simulink model "Assignment_II_simulink"  (R2024b)
settings: Solver=FixedStepAuto  StartTime=0.0  StopTime=inf  FixedStep=1/f_cmd  RelTol=1e-3
values from neighbouring files (symbols this model uses):
  ang_max = 0.05    [Assignment_II.m]
  dist_max = 0.01    [Assignment_II.m]
  k_v = 3    [Assignment_II.m]
  k_w_direction = 3    [Assignment_II.m]
  k_w_heading = 1    [Assignment_II.m]
  turtlebot3 = [ ... (first row only)    [Assignment_II.m]
  v_max = 0.2    [Assignment_II.m]
  yaw_rate_max = 0.4    [Assignment_II.m]
undefined symbols (not defined in the file or in its folder): Angular, Linear
libraries: robotlib x3, simulink x2
settings Model: PacingRate=20  Creator=vigno  LastModifiedBy=vigno
settings OptimizationCC: EnhancedBackFolding=on  PassReuseOutputArgsAs=Individual arguments  ZeroExternalMemoryAtStartup=off  ZeroInternalMemoryAtStartup=off  MaxStackSize=64  OptimizeBlockOrder=speed  DifferentSizesBufferReuse=on  OptimizationCustomize=off  EfficientTunableParamExpr=on
settings DebuggingCC: ParameterTunabilityLossMsg=error
settings HardwareCC: ProdBitPerPointer=32  ProdBitPerSizeT=32  ProdBitPerPtrDiffT=32  ProdLargestAtomicFloat=None  ProdIntDivRoundTo=Undefined  ProdEndianess=Unspecified  ProdWordSize=32  ProdHWDeviceType=Generic->Unspecified (assume 32-bit Generic)
settings ModelReferenceCC: EnableRefExpFcnMdlSchedulingChecks=on
settings SFSimCC: MATLABDynamicMemAlloc=off
settings RTWCC: Description=Embedded Coder  SystemTargetFile=ert.tlc  HardwareBoard=Robot Operating System (ROS)  TLCOptions="-aInlineSetEventsForThisBaseRateFcn=TLC_FALSE -aSuppressMultiTaskScheduler=TLC_FALSE  -aRateBasedStepFcn=0"  TemplateMakefile=ert_default_tmf  Toolchain=Catkin  TargetLang=C++  GPUComputeCapability=3.5
settings CodeAppCC: ForceParamTrailComments=on  IgnoreCustomStorageClasses=off  OperatorAnnotations=on  SimulinkDataObjDesc=on  SFDataObjDesc=on  InsertBlockDesc=on
settings ERTTargetCC: InlinedParameterPlacement=Hierarchical  DynamicArrayContainerType=coder::array

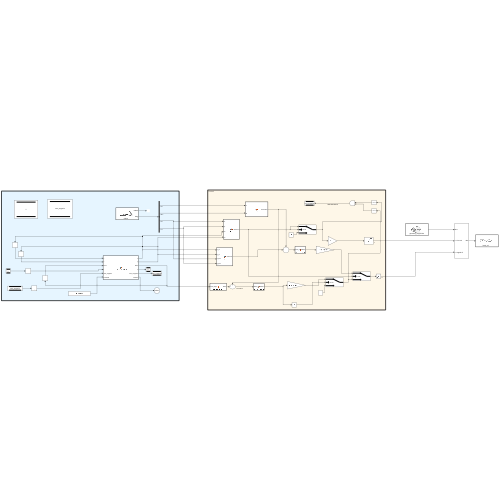
[thumbnail: Simulink's stored preview of the top-level diagram]
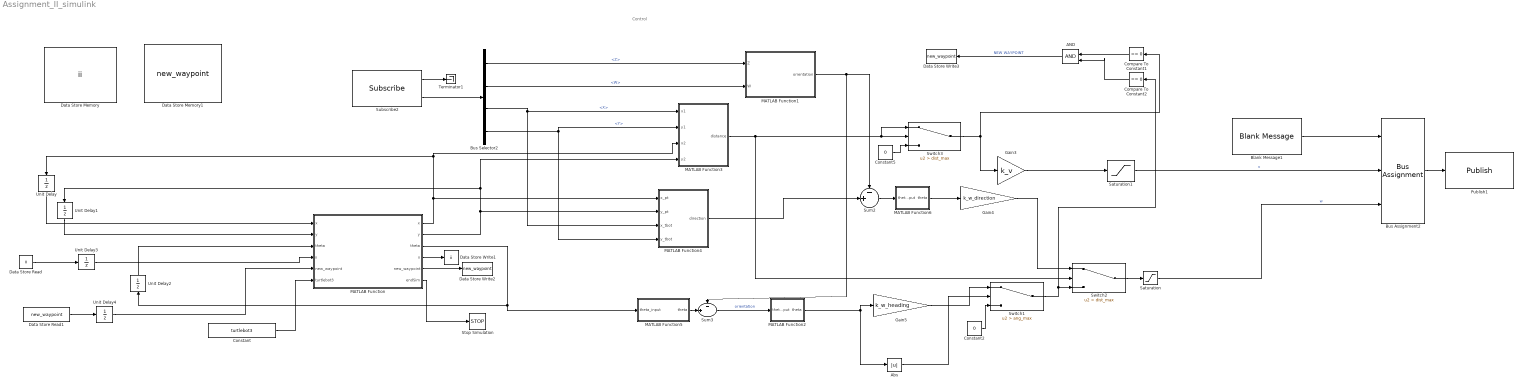
== system Assignment_II_simulink ==
  note: Control
  AND : Logic  IconShape=distinctive  AllPortsSameDT=off  OutDataTypeStr=boolean
  Abs : Abs  SaturateOnIntegerOverflow=off
  Blank Message1 : robotlib/Blank Message  messageClass=Message  entityType=geometry_msgs/Twist  messageType=geometry_msgs/Twist  SampleTime=-1  legacyBusStruct=off
  Bus Assignment2 : BusAssignment  AssignedSignals=Linear.X,Angular.Z
  Bus Selector2 : BusSelector  OutputSignals=Pose.Pose.Orientation.Z,Pose.Pose.Orientation.W,Pose.Pose.Position.X,Pose.Pose.Position.Y
  Compare To Constant1 : simulink/Logic and Bit Operations/Compare To Constant  relop===  const=0  OutDataTypeStr=boolean
  Compare To Constant2 : simulink/Logic and Bit Operations/Compare To Constant  relop===  const=0  OutDataTypeStr=boolean
  Constant : Constant  Value=turtlebot3
  Constant2 : Constant  Value=0
  Constant5 : Constant  Value=0
  Data Store Memory : DataStoreMemory  DataStoreName=ii  WriteAfterWriteMsg=warning  ShowAdditionalParam=off  OutDataTypeStr=double
  Data Store Memory1 : DataStoreMemory  DataStoreName=new_waypoint  WriteAfterWriteMsg=warning  ShowAdditionalParam=off
  Data Store Read : DataStoreRead  DataStoreName=ii  IndexOptions=Index vector (dialog)  Indices=1  OutputSizes=1
  Data Store Read1 : DataStoreRead  DataStoreName=new_waypoint  IndexOptions=Index vector (dialog)  Indices=1  OutputSizes=1
  Data Store Write1 : DataStoreWrite  DataStoreName=ii  IndexOptions=Index vector (dialog)  Indices=1  OutputSizes=1
  Data Store Write2 : DataStoreWrite  DataStoreName=new_waypoint  IndexOptions=Index vector (dialog)  Indices=1  OutputSizes=1
  Data Store Write3 : DataStoreWrite  DataStoreName=new_waypoint  IndexOptions=Index vector (dialog)  Indices=1  OutputSizes=1
  Gain3 : Gain  Gain=k_v
  Gain4 : Gain  Gain=k_w_direction
  Gain5 : Gain  Gain=k_w_heading
  MATLAB Function : MATLAB Function  TreatAsAtomicUnit=on
  MATLAB Function1 : MATLAB Function  TreatAsAtomicUnit=on
  MATLAB Function2 : MATLAB Function  TreatAsAtomicUnit=on
  MATLAB Function3 : MATLAB Function  TreatAsAtomicUnit=on
  MATLAB Function4 : MATLAB Function  TreatAsAtomicUnit=on
  MATLAB Function5 : MATLAB Function  TreatAsAtomicUnit=on
  MATLAB Function6 : MATLAB Function  TreatAsAtomicUnit=on
  Publish1 : robotlib/Publish  topicSource=Select from ROS network  topic=/cmd_vel  messageType=geometry_msgs/Twist  legacyBusStruct=off  messageQueueLength=1
  Saturation : Saturate  UpperLimit=yaw_rate_max  LowerLimit=- yaw_rate_max
  Saturation1 : Saturate  UpperLimit=v_max  LowerLimit=- v_max
  Stop Simulation : Stop
  Subscribe2 : robotlib/Subscribe  topicSource=Select from ROS network  topic=/odom  messageType=nav_msgs/Odometry  SampleTime=-1  legacyBusStruct=off  messageQueueLength=1
  Sum2 : Sum  Inputs=-+|
  Sum3 : Sum  Inputs=-+|
  Switch1 : Switch  Criteria=u2 > Threshold  Threshold=ang_max  SaturateOnIntegerOverflow=off  InputSameDT=off
  Switch2 : Switch  Criteria=u2 > Threshold  Threshold=dist_max  SaturateOnIntegerOverflow=off  InputSameDT=off
  Switch3 : Switch  Criteria=u2 > Threshold  Threshold=dist_max  SaturateOnIntegerOverflow=off  InputSameDT=off
  Terminator1 : Terminator
  Unit Delay{,1..4} (5 alike) : UnitDelay  SampleTime=-1  HasFrameUpgradeWarning=on
  wires:
  Subscribe2/2 -> Bus Selector2/1
  Blank Message1/1 -> Bus Assignment2/1
  Switch3/1 -> Compare To Constant1/1, Gain3/1
  Bus Selector2/2 -> MATLAB Function1/2(W)  "<W>"
  Gain3/1 -> Saturation1/1
  Bus Assignment2/1 -> Publish1/1
  Subscribe2/1 -> Terminator1/1
  Gain4/1 -> Switch2/1
  MATLAB Function4/1(direction) -> Sum2/2
  MATLAB Function3/1(distance) -> Switch3/1, Switch3/2, Switch2/2
  Constant5/1 -> Switch3/3
  Sum3/1 -> MATLAB Function2/1(theta_input)  "orientation"
  MATLAB Function1/1(orientation) -> Sum2/1, Sum3/1
  Bus Selector2/4 -> MATLAB Function3/2(y1), MATLAB Function4/4(y_tbot)  "<Y>"
  Bus Selector2/1 -> MATLAB Function1/1(Z)  "<Z>"
  Sum2/1 -> MATLAB Function6/1(theta_input)
  Bus Selector2/3 -> MATLAB Function4/3(x_tbot), MATLAB Function3/1(x1)  "<X>"
  AND/1 -> Data Store Write3/1  "NEW WAYPOINT"
  Data Store Read/1 -> Unit Delay3/1
  Data Store Read1/1 -> Unit Delay4/1
  MATLAB Function/2(y) -> MATLAB Function4/2(y_pt), MATLAB Function3/4(y2), Unit Delay1/1
  MATLAB Function/1(x) -> MATLAB Function4/1(x_pt), MATLAB Function3/3(x2), Unit Delay/1
  MATLAB Function/4(ii) -> Data Store Write1/1
  MATLAB Function/5(new_waypoint) -> Data Store Write2/1
  MATLAB Function/6(endSim) -> Stop Simulation/1
  Constant/1 -> MATLAB Function/6(turtlebot3)
  Unit Delay/1 -> MATLAB Function/1("x ")
  Unit Delay1/1 -> MATLAB Function/2("y ")
  Unit Delay2/1 -> MATLAB Function/3("theta ")
  Unit Delay3/1 -> MATLAB Function/4("ii ")
  Unit Delay4/1 -> MATLAB Function/5("new_waypoint ")
  Compare To Constant2/1 -> AND/2
  Compare To Constant1/1 -> AND/1
  Constant2/1 -> Switch1/3
  Switch1/1 -> Compare To Constant2/1, Switch2/3
  Gain5/1 -> Switch1/1
  MATLAB Function/3(theta) -> MATLAB Function5/1(theta_input), Unit Delay2/1
  Abs/1 -> Switch1/2
  MATLAB Function5/1(theta) -> Sum3/2
  MATLAB Function2/1(theta) -> Abs/1, Gain5/1
  Switch2/1 -> Saturation/1
  MATLAB Function6/1(theta) -> Gain4/1
  Saturation/1 -> Bus Assignment2/3  "w"
  Saturation1/1 -> Bus Assignment2/2  "v"

== matlab function Assignment_II_simulink/MATLAB Function2 ==
  data: theta_input input; theta output
function theta = correct_angle(theta_input)
    if theta_input <= pi && theta_input >= -pi
        theta = theta_input;
    else
        theta = mod(theta_input + pi, 2 * pi) - pi;
    end
end

== matlab function Assignment_II_simulink/MATLAB Function ==
  data: x input; y input; theta input; ii input; x output; y output; new_waypoint input; theta output; ii output; new_waypoint output; turtlebot3 input; endSim output
function [x, y, theta, ii, new_waypoint, endSim] = new_waypointer(x, y, theta, ii, new_waypoint, turtlebot3)
    endSim = false;
    if new_waypoint
        ii = double(ii);
        ii = ii + 1;
        if ii > size(turtlebot3, 1)
            endSim = true;
            return
        else
            x = turtlebot3(ii, 1);
            y = turtlebot3(ii, 2);
            theta = turtlebot3(ii, 3);
        end
    end
end

== matlab function Assignment_II_simulink/MATLAB Function5 ==
  data: theta_input input; theta output
function theta = correct_angle(theta_input)
    if theta_input <= pi && theta_input >= -pi
        theta = theta_input;
    else
        theta = mod(theta_input + pi, 2 * pi) - pi;
    end
end

== matlab function Assignment_II_simulink/MATLAB Function6 ==
  data: theta_input input; theta output
function theta = correct_angle(theta_input)
    if theta_input <= pi && theta_input >= -pi
        theta = theta_input;
    else
        theta = mod(theta_input + pi, 2 * pi) - pi;
    end
end

== matlab function Assignment_II_simulink/MATLAB Function1 ==
  data: Z input; orientation output; W input
function orientation = fcn(Z, W)
    orientation = 2 * atan2(Z, W);
    if orientation > pi
        orientation = orientation - 2 * pi;
    elseif orientation < -pi
        orientation = orientation + 2 * pi;
    end
end

== matlab function Assignment_II_simulink/MATLAB Function3 ==
  data: x1 input; distance output; y1 input; x2 input; y2 input
function distance = fcn(x1, y1, x2, y2)
    distance = sqrt((x1 - x2)^2 + (y1 - y2)^2);

== matlab function Assignment_II_simulink/MATLAB Function4 ==
  data: x_pt input; direction output; y_pt input; x_tbot input; y_tbot input
function direction = fcn(x_pt, y_pt, x_tbot, y_tbot)
    direction = atan2(y_pt - y_tbot, x_pt - x_tbot);
